simulink model "Step_7_Data_Extraction_2"  (R2020a)
settings: Solver=ode3  StartTime=0.0  StopTime=10.0  FixedStep=0.001  RelTol=1e-3  EnableMultiTasking=on
settings Model: Creator=i7  LastModifiedBy=nnnmmm
settings DataIOCC: LimitDataPoints=on  SaveFormat=Array  ReturnWorkspaceOutputs=off
settings OptimizationCC: ExpressionDepthLimit=2147483647  LifeSpan=inf
settings DebuggingCC: UnderspecifiedInitializationDetection=Classic  MergeDetectMultiDrivingBlocksExec=none  SolverPrmCheckMsg=warning  FcnCallInpInsideContextMsg=warning  StateNameClashWarn=warning  SFUnexpectedBacktrackingDiag=warning  SFNoUnconditionalDefaultTransitionDiag=warning  SFExecutionAtInitializationDiag=none  ArithmeticOperatorsInVariantConditions=warning
settings HardwareCC: ProdBitPerPointer=32  ProdBitPerSizeT=32  ProdBitPerPtrDiffT=32  ProdLargestAtomicFloat=None  ProdIntDivRoundTo=Undefined  ProdEndianess=Unspecified  ProdWordSize=32  ProdHWDeviceType=32-bit Generic
settings ModelReferenceCC: PropagateSignalLabelsOutOfModel=off
settings SFSimCC: SimUseLocalCustomCode=off  CustomCodeUndefinedFunction=UseInterfaceOnly
settings RTWCC: RTWUseLocalCustomCode=off
settings CodeAppCC: StateflowObjectComments=on
settings GRTTargetCC: TargetLangStandard=C89/C90 (ANSI)  CombineOutputUpdateFcns=off  GRTInterface=on
settings ConfigComp: CovMetricSettings=dw  CovHtmlReporting=on  CovSaveCumulativeToWorkspaceVar=on  CovSaveSingleToWorkspaceVar=on  CovExternalEMLEnable=off

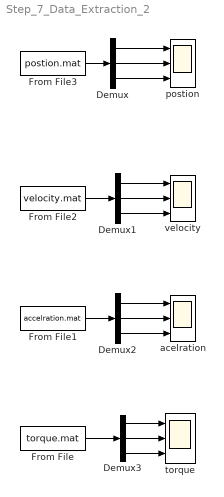
== system Step_7_Data_Extraction_2 ==
  Demux{,1..3} (4 alike) : Demux  Outputs=3
  From File : FromFile  FileName=torque.mat  SampleTime=0
  From File1 : FromFile  FileName=accelration.mat  SampleTime=0
  From File2 : FromFile  FileName=velocity.mat  SampleTime=0
  From File3 : FromFile  FileName=postion.mat  SampleTime=0
  acelration : Scope  NumInputPorts=3
  postion : Scope  NumInputPorts=3
  torque : Scope  NumInputPorts=3
  velocity : Scope  NumInputPorts=3
  wires:
  Demux/1 -> postion/1
  Demux/2 -> postion/2
  Demux/3 -> postion/3
  Demux1/1 -> velocity/1
  Demux1/2 -> velocity/2
  Demux1/3 -> velocity/3
  Demux2/1 -> acelration/1
  Demux2/2 -> acelration/2
  Demux2/3 -> acelration/3
  Demux3/1 -> torque/1
  Demux3/2 -> torque/2
  Demux3/3 -> torque/3
  From File/1 -> Demux3/1
  From File1/1 -> Demux2/1
  From File2/1 -> Demux1/1
  From File3/1 -> Demux/1
